simulink model "closedloop"  (R2018a)
settings: Solver=FixedStepAuto  StartTime=0.0  StopTime=10  FixedStep=Ts  RelTol=1e-3
values from neighbouring files (symbols this model uses):
  A = [cos(theta) -sin(theta) 0 0;sin(theta) cos(theta) 0 0;0 0 1 0;0 0 0 1]*     [1 0 0 0; 0 1 0 0; 0 0 1 d; 0 0 0 1]*     [1 0 0 a; 0 1 0 0; 0 0 1 0; 0 0 0 1]*     [1 0 0 0; 0 0 1 0;0 -1 0 0;0 0 0 1]    [DE_Generator.m]    (also in GUI_ellipsoid.m = [0 1; 0 0]; question3.m = double(subs(DziDzj)); question4.m = [])
  B = [0; 1]    [GUI_ellipsoid.m]    (also in question3.m = double(subs(DziDuj)); question4.m)
  K = handles.K    [GUI_ellipsoid.m]    (also in question3.m = lqr(A, B, Q, R); question4.m = dlqr(Ad, Bd, diag([100 1]),0.1); waterheater.m = inv(G'*Q*G + R*eye*(Nm))*G')
  Kdb = place(Ak,Bk,rand(8,1)*1e-5)    [question3.m]
  Kk = dlqr(Ak, Bk, Q, R)    [question3.m]
  Ts = 0.01    [GUI_ellipsoid.m]    (also in question3.m; question4.m)
  ub = u0    [question3.m]    (also in question4.m = [])
  z0 = zb*1.2    [question3.m]
  zb = z0    [question3.m]
undefined symbols (not defined in the file or in its folder): Ak, Bk, stateder
settings Model: Creator=rhanz  LastModifiedBy=erivelton

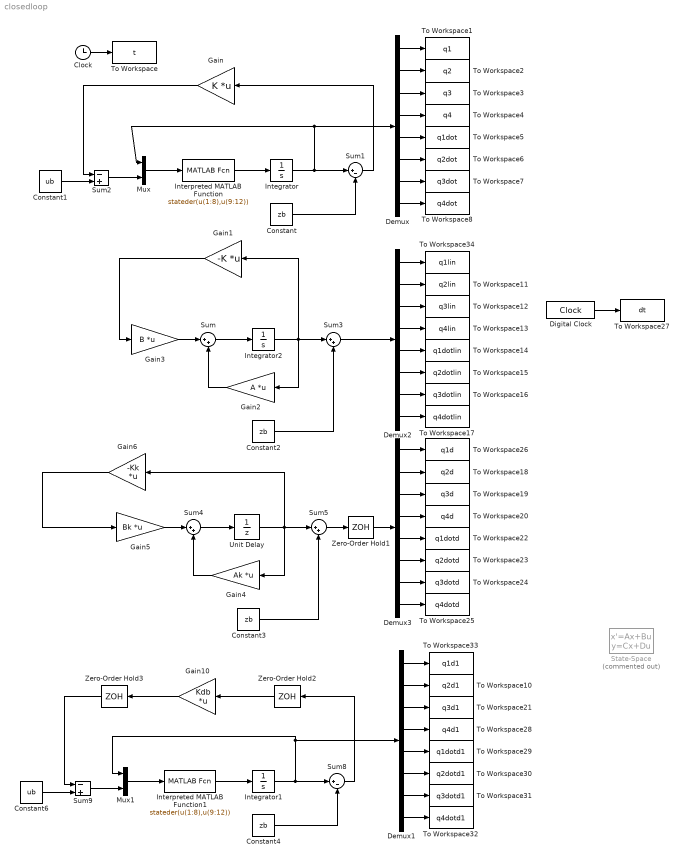
== system closedloop ==
  Clock : Clock
  Constant{,2..4} (4 alike) : Constant  Value=zb
  Constant1 : Constant  Value=ub
  Constant6 : Constant  Value=ub
  Demux{,1..3} (4 alike) : Demux  Outputs=8
  Digital Clock : DigitalClock  SampleTime=Ts
  Gain : Gain  Gain=K  Multiplication=Matrix(K*u) (u vector)
  Gain1 : Gain  Gain=-K  Multiplication=Matrix(K*u) (u vector)
  Gain10 : Gain  Gain=Kdb  Multiplication=Matrix(K*u) (u vector)
  Gain2 : Gain  Gain=A  Multiplication=Matrix(K*u) (u vector)
  Gain3 : Gain  Gain=B  Multiplication=Matrix(K*u) (u vector)
  Gain4 : Gain  Gain=Ak  Multiplication=Matrix(K*u) (u vector)
  Gain5 : Gain  Gain=Bk  Multiplication=Matrix(K*u) (u vector)
  Gain6 : Gain  Gain=-Kk  Multiplication=Matrix(K*u) (u vector)
  Integrator : Integrator  InitialCondition=z0+zb
  Integrator1 : Integrator  InitialCondition=z0
  Integrator2 : Integrator  InitialCondition=z0
  Interpreted MATLAB Function : MATLABFcn  MATLABFcn=stateder(u(1:8),u(9:12))  OutputDimensions=8
  Interpreted MATLAB Function1 : MATLABFcn  MATLABFcn=stateder(u(1:8),u(9:12))  OutputDimensions=8
  Mux : Mux  Inputs=2
  Mux1 : Mux  Inputs=2
  State-Space : StateSpace  Commented=on  A=A  B=B  C=eye(8)  D=zeros(8,4)  InitialCondition=0
  Sum{,3..5} (4 alike) : Sum  Inputs=|++
  Sum1 : Sum  Inputs=|+-
  Sum2 : Sum  Inputs=-+
  Sum8 : Sum  Inputs=|+-
  Sum9 : Sum  Inputs=-+
  To Workspace : ToWorkspace  VariableName=t  SampleTime=-1
  To Workspace1 : ToWorkspace  VariableName=q1  SampleTime=-1
  To Workspace10 : ToWorkspace  VariableName=q2d1  SampleTime=-1
  To Workspace11 : ToWorkspace  VariableName=q2lin  SampleTime=-1
  To Workspace12 : ToWorkspace  VariableName=q3lin  SampleTime=-1
  To Workspace13 : ToWorkspace  VariableName=q4lin  SampleTime=-1
  To Workspace14 : ToWorkspace  VariableName=q1dotlin  SampleTime=-1
  To Workspace15 : ToWorkspace  VariableName=q2dotlin  SampleTime=-1
  To Workspace16 : ToWorkspace  VariableName=q3dotlin  SampleTime=-1
  To Workspace17 : ToWorkspace  VariableName=q4dotlin  SampleTime=-1
  To Workspace18 : ToWorkspace  VariableName=q2d  SampleTime=-1
  To Workspace19 : ToWorkspace  VariableName=q3d  SampleTime=-1
  To Workspace2 : ToWorkspace  VariableName=q2  SampleTime=-1
  To Workspace20 : ToWorkspace  VariableName=q4d  SampleTime=-1
  To Workspace21 : ToWorkspace  VariableName=q3d1  SampleTime=-1
  To Workspace22 : ToWorkspace  VariableName=q1dotd  SampleTime=-1
  To Workspace23 : ToWorkspace  VariableName=q2dotd  SampleTime=-1
  To Workspace24 : ToWorkspace  VariableName=q3dotd  SampleTime=-1
  To Workspace25 : ToWorkspace  VariableName=q4dotd  SampleTime=-1
  To Workspace26 : ToWorkspace  VariableName=q1d  SampleTime=-1
  To Workspace27 : ToWorkspace  VariableName=dt  SampleTime=-1
  To Workspace28 : ToWorkspace  VariableName=q4d1  SampleTime=-1
  To Workspace29 : ToWorkspace  VariableName=q1dotd1  SampleTime=-1
  To Workspace3 : ToWorkspace  VariableName=q3  SampleTime=-1
  To Workspace30 : ToWorkspace  VariableName=q2dotd1  SampleTime=-1
  To Workspace31 : ToWorkspace  VariableName=q3dotd1  SampleTime=-1
  To Workspace32 : ToWorkspace  VariableName=q4dotd1  SampleTime=-1
  To Workspace33 : ToWorkspace  VariableName=q1d1  SampleTime=-1
  To Workspace34 : ToWorkspace  VariableName=q1lin  SampleTime=-1
  To Workspace4 : ToWorkspace  VariableName=q4  SampleTime=-1
  To Workspace5 : ToWorkspace  VariableName=q1dot  SampleTime=-1
  To Workspace6 : ToWorkspace  VariableName=q2dot  SampleTime=-1
  To Workspace7 : ToWorkspace  VariableName=q3dot  SampleTime=-1
  To Workspace8 : ToWorkspace  VariableName=q4dot  SampleTime=-1
  Unit Delay : UnitDelay  InitialCondition=z0  SampleTime=Ts
  Zero-Order Hold1 : ZeroOrderHold  SampleTime=Ts
  Zero-Order Hold2 : ZeroOrderHold  SampleTime=Ts
  Zero-Order Hold3 : ZeroOrderHold  SampleTime=Ts
  wires:
  Interpreted MATLAB Function/1 -> Integrator/1
  Mux/1 -> Interpreted MATLAB Function/1
  Integrator/1 -> Demux/1, Mux/1, Sum1/1
  Clock/1 -> To Workspace/1
  Demux/1 -> To Workspace1/1
  Demux/2 -> To Workspace2/1
  Demux/3 -> To Workspace3/1
  Demux/4 -> To Workspace4/1
  Demux/5 -> To Workspace5/1
  Demux/6 -> To Workspace6/1
  Demux/7 -> To Workspace7/1
  Demux/8 -> To Workspace8/1
  Constant/1 -> Sum1/2
  Sum2/1 -> Mux/2
  Gain/1 -> Sum2/1
  Constant1/1 -> Sum2/2
  Demux3/5 -> To Workspace22/1
  Demux2/8 -> To Workspace17/1
  Demux3/7 -> To Workspace24/1
  Demux2/3 -> To Workspace12/1
  Demux3/4 -> To Workspace20/1
  Demux2/1 -> To Workspace34/1
  Constant2/1 -> Sum3/2
  Sum3/1 -> Demux2/1
  Demux3/6 -> To Workspace23/1
  Demux2/2 -> To Workspace11/1
  Integrator2/1 -> Gain1/1, Sum3/1, Gain2/1
  Demux2/7 -> To Workspace16/1
  Zero-Order Hold1/1 -> Demux3/1
  Demux2/4 -> To Workspace13/1
  Sum4/1 -> Unit Delay/1
  Gain6/1 -> Gain5/1
  Demux3/3 -> To Workspace19/1
  Constant3/1 -> Sum5/2
  Demux3/8 -> To Workspace25/1
  Sum5/1 -> Zero-Order Hold1/1
  Gain3/1 -> Sum/1
  Gain4/1 -> Sum4/2
  Gain2/1 -> Sum/2
  Demux2/6 -> To Workspace15/1
  Demux3/2 -> To Workspace18/1
  Demux3/1 -> To Workspace26/1
  Gain5/1 -> Sum4/1
  Digital Clock/1 -> To Workspace27/1
  Demux2/5 -> To Workspace14/1
  Sum/1 -> Integrator2/1
  Gain1/1 -> Gain3/1
  Unit Delay/1 -> Gain6/1, Sum5/1, Gain4/1
  Demux1/2 -> To Workspace10/1
  Demux1/8 -> To Workspace32/1
  Demux1/6 -> To Workspace30/1
  Demux1/4 -> To Workspace28/1
  Integrator1/1 -> Demux1/1, Mux1/1, Sum8/1
  Demux1/7 -> To Workspace31/1
  Demux1/5 -> To Workspace29/1
  Demux1/1 -> To Workspace33/1
  Demux1/3 -> To Workspace21/1
  Gain10/1 -> Zero-Order Hold3/1
  Constant6/1 -> Sum9/2
  Sum9/1 -> Mux1/2
  Interpreted MATLAB Function1/1 -> Integrator1/1
  Mux1/1 -> Interpreted MATLAB Function1/1
  Sum8/1 -> Zero-Order Hold2/1
  Constant4/1 -> Sum8/2
  Zero-Order Hold2/1 -> Gain10/1
  Zero-Order Hold3/1 -> Sum9/1
  Sum1/1 -> Gain/1
